simulink model "rule_intersection"  (R2021a)
settings: Solver=FixedStepAuto  StartTime=0.0  StopTime=47  FixedStep=0.1  RelTol=1e-3
values from neighbouring files (symbols this model uses):
  Cross =     [Cross.mat]
libraries: simulink x17
(part 2 of 2)

== matlab function rule_intersection/right of way/红灯右转路权监测/Enabled Subsystem/stage2/MATLAB Function1 ==
  data: Decision_A_x input; Decision_A_y input; Tgt input; y output; Ego input; Thetamin input; Thetamax input
function y = fcn(Decision_A_x,Decision_A_y,Tgt,Ego,Thetamin,Thetamax)
Tgtx = Tgt.TgtX;
Tgty = Tgt.TgtY;
Tgttheta = Tgt.Tgttheta;
Egovx = Ego.Egovx;
flag = (Tgttheta>Thetamin(1) & Tgttheta<Thetamax(1)) | (Tgttheta>Thetamin(2) & Tgttheta<Thetamax(2));
Tgtx = Tgtx.*flag;
Tgty = Tgty.*flag;
[in,~] = inpolygon(Tgtx,Tgty,Decision_A_x,Decision_A_y);

if sum(in)>0 && Egovx==0
    y = 1;
else
    y = 0;
end

== matlab function rule_intersection/right of way/左转路权监测/对向直行车道交点/rightarc_r ==
  data: u1 input; X output; u2 input; Y output; u4 input; u6 input
function [X,Y] = fcn(u1,u2,u4,u6)

locate_rf = [u1(7),u1(8)];
intention_rr = [u2(7),u2(8)];
r2l1_rf = [u4(5),u4(6)];
r4l_1_rr = [u6(7),u6(8)];
[x1,y1] = arc_generate_l(locate_rf(1),locate_rf(2),intention_rr(1),intention_rr(2));
for i = 1:19
    X1 = [x1(i),y1(i)]; X2 = [x1(i+1),y1(i+1)];
    [y,X,Y] = iscross(r2l1_rf,r4l_1_rr,X1,X2);
    if y == 1
        break
    end
end

== matlab function rule_intersection/right of way/左转路权监测/对向直行车道交点/MATLAB Function ==
  data: r_1r input; Intersect_A_x output; r_1l input; l_1r input; l_1l input; DPl input; DPr input; Intersect_A_y output; Decision_A_x output; Decision_A_y output
function [Intersect_A_x,Intersect_A_y,Decision_A_x,Decision_A_y] = fcn(r_1r,r_1l,l_1r,l_1l,DPl,DPr)

Intersect_A_x = [r_1r(1),r_1l(1),l_1l(1),l_1r(1),r_1r(1)];
Intersect_A_y = [r_1r(2),r_1l(2),l_1l(2),l_1r(2),r_1r(2)];
Decision_A_x = [l_1r(1),l_1l(1),DPl(1),DPr(1),l_1r(1)];
Decision_A_y = [l_1r(2),l_1l(2),DPl(2),DPr(2),l_1r(2)];

== matlab function rule_intersection/自车五个点 ==
  data: Ego input; X output; Y output
function [X,Y] = fcn(Ego)
Egox = Ego.EgoX;
Egoy = Ego.EgoY;
theta = Ego.Egotheta;
length = Ego.length;
width = Ego.width;
lf_x = Egox + 0.5*length*cos(theta) - 0.5*width*sin(theta);
lf_y = Egoy + 0.5*length*sin(theta) + 0.5*width*cos(theta);
lr_x = Egox - 0.5*length*cos(theta) - 0.5*width*sin(theta);
lr_y = Egoy - 0.5*length*sin(theta) + 0.5*width*cos(theta);
rf_x = Egox + 0.5*length*cos(theta) + 0.5*width*sin(theta);
rf_y = Egoy + 0.5*length*sin(theta) - 0.5*width*cos(theta);
rr_x = Egox - 0.5*length*cos(theta) + 0.5*width*sin(theta);
rr_y = Egoy - 0.5*length*sin(theta) - 0.5*width*cos(theta);
X = [Egox,lf_x,lr_x,rf_x,rr_x];
Y = [Egoy,lf_y,lr_y,rf_y,rr_y];

== matlab function rule_intersection/right of way/左转路权监测/MATLAB Function ==
  data: X input; t1 output; Y input; Intersect_A_x input; Intersect_A_y input; t2 output
function [t1,t2] = fcn(X,Y,Intersect_A_x,Intersect_A_y)
[in1,~] = inpolygon(X(1),Y(1),Intersect_A_x,Intersect_A_y);
[in2,~] = inpolygon(X(2),Y(2),Intersect_A_x,Intersect_A_y);
if ~in1 & in2  %驶入阶段
    t1 = 1;
    t2 = 0;
elseif in1  %通过阶段
    t1 = 0;
    t2 = 1;
else
    t1 = 0;
    t2 = 0;
end

== matlab function rule_intersection/right of way/Subsystem/MATLAB Function1 ==
  data: u input; y output
function y = fcn(u)

y = sign(u(1));

== matlab function rule_intersection/right of way/左转路权监测/输出对向方向预测线 ==
  data: u input; DPline output; Cross input; Theta_max output; Theta_min output
function [DPline,Theta_max,Theta_min] = fcn(u,Cross)

if u(1) == 1
    Zin = Cross.road3.zin;
    DPline = [Zin(1)+0,Zin(2),Zin(5)+0,Zin(6)];
    Theta_max = [15*pi/180,0];
    Theta_min = [0,-15*pi/180];
elseif u(1) == 2
    Zin = Cross.road4.zin;
    DPline = [Zin(1),Zin(2)+0,Zin(5),Zin(6)+0];
    Theta_max = [105*pi/180,90*pi/180];
    Theta_min = [90*pi/180,75*pi/180];
elseif u(1) == 3
    Zin = Cross.road1.zin;
    DPline = [Zin(1)-0,Zin(2),Zin(5)-0,Zin(6)];
    Theta_max = [pi,-165*pi/180];
    Theta_min = [165*pi/180,-pi];
else
    Zin = Cross.road2.zin;
    DPline = [Zin(1),Zin(2)-0,Zin(5),Zin(6)-0];
    Theta_max = [-75*pi/180,-90*pi/180];
    Theta_min = [-90*pi/180,-105*pi/180];
end

== matlab function rule_intersection/right of way/红灯右转路权监测/MATLAB Function ==
  data: X input; t1 output; Y input; Intersect_A_x input; Intersect_A_y input; t2 output
function [t1,t2] = fcn(X,Y,Intersect_A_x,Intersect_A_y)
[in1,~] = inpolygon(X(1),Y(1),Intersect_A_x,Intersect_A_y);
[in2,~] = inpolygon(X(2),Y(2),Intersect_A_x,Intersect_A_y);
if ~in1 & in2  %驶入阶段
    t1 = 1;
    t2 = 0;
elseif in1  %通过阶段
    t1 = 0;
    t2 = 1;
else
    t1 = 0;
    t2 = 0;
end

== matlab function rule_intersection/right of way/红灯右转路权监测/左侧直行车道交点/DPline_直行交点 ==
  data: u1 input; u3 input; u4 input; u5 input; u6 input; r2l1_DP_l output; u input; r2l1_DP_r output
function [r2l1_DP_l,r2l1_DP_r] = fcn(u1,u3,u4,u5,u6,u)

DPline_l = [u(1),u(2)];
DPline_r = [u(3),u(4)];

r2l1_lf = [u3(1),u3(2)];
r4l_1_lr = [u5(3),u5(4)];
r2l1_rf = [u4(5),u4(6)];
r4l_1_rr = [u6(7),u6(8)];
[~,Xl,Yl] = iscross(r2l1_lf,r4l_1_lr,DPline_l,DPline_r);
[~,Xr,Yr] = iscross(r2l1_rf,r4l_1_rr,DPline_l,DPline_r);
r2l1_DP_l = [Xl,Yl];
r2l1_DP_r = [Xr,Yr];

== matlab function rule_intersection/right of way/红灯右转路权监测/左侧直行车道交点/MATLAB Function ==
  data: r_r input; Intersect_A_x output; r_l input; l_r input; l_l input; DPl input; DPr input; Intersect_A_y output; Decision_A_x output; Decision_A_y output
function [Intersect_A_x,Intersect_A_y,Decision_A_x,Decision_A_y] = fcn(r_r,r_l,l_r,l_l,DPl,DPr)

Intersect_A_x = [r_r(1),r_l(1),l_l(1),l_r(1),r_r(1)];
Intersect_A_y = [r_r(2),r_l(2),l_l(2),l_r(2),r_r(2)];
Decision_A_x = [l_r(1),l_l(1),DPl(1),DPr(1),l_r(1)];
Decision_A_y = [l_r(2),l_l(2),DPl(2),DPr(2),l_r(2)];

== matlab function rule_intersection/right of way/红灯右转路权监测/左侧直行车道交点/leftarc_l ==
  data: u1 input; X output; u2 input; Y output; u3 input; u5 input
function [X,Y] = fcn(u1,u2,u3,u5)

locate_lf = [u1(3),u1(4)];
intention_lr = [u2(3),u2(4)];
r2l1_lf = [u3(1),u3(2)];
r4l_1_lr = [u5(3),u5(4)];
[x1,y1] = arc_generate_r(locate_lf(1),locate_lf(2),intention_lr(1),intention_lr(2));
x1 = [intention_lr(1),x1(2:end)];
y1 = [intention_lr(2),y1(2:end)];
for i = 1:19
    X1 = [x1(i),y1(i)]; X2 = [x1(i+1),y1(i+1)];
    [y,X,Y] = iscross(r2l1_lf,r4l_1_lr,X1,X2);
    if y == 1
        break
    end
end

== matlab function rule_intersection/right of way/左转路权监测/对向直行车道交点/DPline_直行交点 ==
  data: u1 input; u3 input; u4 input; u5 input; u6 input; r2l1_DP_l output; u input; r2l1_DP_r output
function [r2l1_DP_l,r2l1_DP_r] = fcn(u1,u3,u4,u5,u6,u)

DPline_l = [u(1),u(2)];
DPline_r = [u(3),u(4)];

r2l1_lf = [u3(1),u3(2)];
r4l_1_lr = [u5(3),u5(4)];
r2l1_rf = [u4(5),u4(6)];
r4l_1_rr = [u6(7),u6(8)];
[~,Xl,Yl] = iscross(r2l1_lf,r4l_1_lr,DPline_l,DPline_r);
[~,Xr,Yr] = iscross(r2l1_rf,r4l_1_rr,DPline_l,DPline_r);
r2l1_DP_l = [Xl,Yl];
r2l1_DP_r = [Xr,Yr];

== matlab function rule_intersection/right of way/红灯右转路权监测/左侧直行车道交点/leftarc_r ==
  data: u1 input; X output; u2 input; Y output; u4 input; u6 input
function [X,Y] = fcn(u1,u2,u4,u6)

locate_lf = [u1(3),u1(4)];
intention_lr = [u2(3),u2(4)];
r2l1_rf = [u4(5),u4(6)];
r4l_1_rr = [u6(7),u6(8)];
[x1,y1] = arc_generate_r(locate_lf(1),locate_lf(2),intention_lr(1),intention_lr(2));
for i = 1:19
    X1 = [x1(i),y1(i)]; X2 = [x1(i+1),y1(i+1)];
    [y,X,Y] = iscross(r2l1_rf,r4l_1_rr,X1,X2);
    if y == 1
        break
    end
end

== matlab function rule_intersection/right of way/左转路权监测/对向直行车道交点/rightarc_l ==
  data: u1 input; X output; u2 input; Y output; u3 input; u5 input
function [X,Y] = fcn(u1,u2,u3,u5)

locate_rf = [u1(7),u1(8)];
intention_rr = [u2(7),u2(8)];
r2l1_lf = [u3(1),u3(2)];
r4l_1_lr = [u5(3),u5(4)];
[x1,y1] = arc_generate_l(locate_rf(1),locate_rf(2),intention_rr(1),intention_rr(2));
for i = 1:19
    X1 = [x1(i),y1(i)]; X2 = [x1(i+1),y1(i+1)];
    [y,X,Y] = iscross(r2l1_lf,r4l_1_lr,X1,X2);
    if y == 1
        break
    end
end

== matlab function rule_intersection/right of way/左转路权监测/Enabled Subsystem/stage2/MATLAB Function1 ==
  data: Decision_A_x input; Decision_A_y input; Tgt input; y output; Ego input; Thetamin input; Thetamax input
function y = fcn(Decision_A_x,Decision_A_y,Tgt,Ego,Thetamin,Thetamax)
Tgtx = Tgt.TgtX;
Tgty = Tgt.TgtY;
Tgttheta = Tgt.Tgttheta;
Egovx = Ego.Egovx;
flag = (Tgttheta>Thetamin(1) & Tgttheta<Thetamax(1)) | (Tgttheta>Thetamin(2) & Tgttheta<Thetamax(2));
Tgtx = Tgtx.*flag;
Tgty = Tgty.*flag;
[in,~] = inpolygon(Tgtx,Tgty,Decision_A_x,Decision_A_y);

if sum(in)>0 && Egovx==0
    y = 1;
else
    y = 0;
end

== matlab function rule_intersection/right of way/红灯右转路权监测/左侧直行车道交点/rightarc_r ==
  data: u1 input; X output; u2 input; Y output; u4 input; u6 input
function [X,Y] = fcn(u1,u2,u4,u6)

locate_rf = [u1(7),u1(8)];
intention_rr = [u2(7),u2(8)];
r2l1_rf = [u4(5),u4(6)];
r4l_1_rr = [u6(7),u6(8)];
[x1,y1] = arc_generate_r(locate_rf(1),locate_rf(2),intention_rr(1),intention_rr(2));
for i = 1:19
    X1 = [x1(i),y1(i)]; X2 = [x1(i+1),y1(i+1)];
    [y,X,Y] = iscross(r2l1_rf,r4l_1_rr,X1,X2);
    if y == 1
        break
    end
end

== matlab function rule_intersection/right of way/红灯右转路权监测/输出左侧方向预测线 ==
  data: u input; DPline output; Cross input; Theta_max output; Theta_min output
function [DPline,Theta_max,Theta_min] = fcn(u,Cross)

if u(1) == 1
    Zin = Cross.road4.zin;
    DPline = [Zin(1),Zin(2)+2,Zin(5),Zin(6)+2];
    Theta_max = [105*pi/180,90*pi/180];
    Theta_min = [90*pi/180,75*pi/180];
elseif u(1) == 2
    Zin = Cross.road1.zin;
    DPline = [Zin(1)-2,Zin(2),Zin(5)-2,Zin(6)];
    Theta_max = [pi,-165*pi/180];
    Theta_min = [165*pi/180,-pi];
elseif u(1) == 3
    Zin = Cross.road2.zin;
    DPline = [Zin(1),Zin(2)-2,Zin(5),Zin(6)-2];
    Theta_max = [-75*pi/180,-90*pi/180];
    Theta_min = [-90*pi/180,-105*pi/180];
else
    Zin = Cross.road3.zin;
    DPline = [Zin(1)+2,Zin(2),Zin(5)+2,Zin(6)];
    Theta_max = [15*pi/180,0];
    Theta_min = [0,-15*pi/180];
end

== matlab function rule_intersection/right of way/输出红绿灯信息 ==
  data: u input; Light input; light output
function light = fcn(u,Light)


if u(1) == 1
    light = Light.light1;
elseif u(1) == 2
    light = Light.light2;
elseif u(1) == 3
    light = Light.light3;
elseif u(1) == 4
    light = Light.light4;
else
    light = 0;
end

== matlab function rule_intersection/right of way/绿灯右转路权监测/Enabled Subsystem/stage1/MATLAB Function2 ==
  data: ODA1 input; ODA2 input; Tgt input; y output; Ego input; Thetamin input; Thetamax input
function y = fcn(ODA1,ODA2,Tgt,Ego,Thetamin,Thetamax)
Tgtx = Tgt.TgtX;
Tgty = Tgt.TgtY;
Tgttheta = Tgt.Tgttheta;
Egovx = Ego.Egovx;
flag = (Tgttheta>Thetamin(1) & Tgttheta<Thetamax(1)) | (Tgttheta>Thetamin(2) & Tgttheta<Thetamax(2));
Tgtx = Tgtx.*flag;
Tgty = Tgty.*flag;
[in1,~] = inpolygon(Tgtx,Tgty,ODA1(1,:),ODA1(2,:));
[in2,~] = inpolygon(Tgtx,Tgty,ODA2(1,:),ODA2(2,:));
in = in1.*in2;

if sum(in)>0 && Egovx~=0
    y = 1;
else
    y = 0;
end

== matlab function rule_intersection/right of way/绿灯右转路权监测/Enabled Subsystem/stage2/MATLAB Function1 ==
  data: ODA1 input; ODA2 input; Tgt input; y output; Ego input; Thetamin input; Thetamax input
function y = fcn(ODA1,ODA2,Tgt,Ego,Thetamin,Thetamax)
Tgtx = Tgt.TgtX;
Tgty = Tgt.TgtY;
Tgttheta = Tgt.Tgttheta;
Egovx = Ego.Egovx;
flag = (Tgttheta>Thetamin(1) & Tgttheta<Thetamax(1)) | (Tgttheta>Thetamin(2) & Tgttheta<Thetamax(2));
Tgtx = Tgtx.*flag;
Tgty = Tgty.*flag;
[in1,~] = inpolygon(Tgtx,Tgty,ODA1(1,:),ODA1(2,:));
[in2,~] = inpolygon(Tgtx,Tgty,ODA2(1,:),ODA2(2,:));
in = in1.*in2;
if sum(in)>0 && Egovx==0
    y = 1;
else
    y = 0;
end

== matlab function rule_intersection/right of way/绿灯右转路权监测/MATLAB Function ==
  data: X input; t1 output; Y input; Intersect_A_x input; Intersect_A_y input; t2 output
function [t1,t2] = fcn(X,Y,Intersect_A_x,Intersect_A_y)
[in1,~] = inpolygon(X(1),Y(1),Intersect_A_x,Intersect_A_y);
[in2,~] = inpolygon((X(2)+X(3))/2,(Y(2)+Y(3))/2,Intersect_A_x,Intersect_A_y);
if ~in1 & in2  %驶入阶段
    t1 = 1;
    t2 = 0;
elseif in1  %通过阶段
    t1 = 0;
    t2 = 1;
else
    t1 = 0;
    t2 = 0;
end

== matlab function rule_intersection/right of way/绿灯右转路权监测/左侧直行车道交点/leftarc_l3 ==
  data: X output; arcx input; arcy input; Y output; u1 input; u2 input
function [X,Y] = fcn(arcx,arcy,u1,u2)
[x1,y1] = arc_generate_r(u1(3),u1(4),u2(3),u2(4));
y = 0;
for i = 1:19
    for j = 1:19
        X1 = [arcx(j),arcy(j)]; X2 = [arcx(j+1),arcy(j+1)];
        X3 = [x1(i),y1(i)]; X4 = [x1(i+1),y1(i+1)];
        [y,X,Y] = iscross(X1,X2,X3,X4);
        if y == 1
            break
        end
    end
    if y == 1
        break
    end
end

== matlab function rule_intersection/virtual lane/Subsystem/MATLAB Function1 ==
  data: u input; y output
function y = fcn(u)

y = sign(u(1));

== matlab function rule_intersection/right of way/绿灯右转路权监测/左侧直行车道交点/MATLAB Function1 ==
  data: u1 input; u2 output; OD_rarc_x output; OD_rarc_y output; ODA1 output; ODA2 output; DPline input
function [u2,OD_rarc_x,OD_rarc_y,ODA1,ODA2] = fcn(u1,DPline)
u2 = zeros(1,11);
u3 = zeros(1,11);
u4 = zeros(1,11);
OD_larc_x = zeros(1,20);
OD_larc_y = zeros(1,20);
OD_rarc_x = zeros(1,20);
OD_rarc_y = zeros(1,20);
coder.extrinsic('tright_G');
[u2,u3,u4] = tright_G(u1);
coder.extrinsic('arc_generate_l')
[OD_larc_x,OD_larc_y]=arc_generate_l(u3(1),u3(2),u2(3),u2(4));
[OD_rarc_x,OD_rarc_y]=arc_generate_l(u4(5),u4(6),u2(7),u2(8));
ODA1 = zeros(2,41);
ODA2 = zeros(2,4);
ODA1(1,:) = [OD_larc_x,fliplr(OD_rarc_x),OD_larc_x(1)];
ODA1(2,:) = [OD_larc_y,fliplr(OD_rarc_y),OD_larc_y(1)];
ODA2(1,:) = [DPline(1:2:5),DPline(1)];
ODA2(2,:) = [DPline(2:2:6),DPline(2)];

== matlab function rule_intersection/right of way/红灯右转路权监测/Enabled Subsystem/stage1/MATLAB Function2 ==
  data: Decision_A_x input; Decision_A_y input; Tgt input; y output; Ego input; Thetamin input; Thetamax input
function y = fcn(Decision_A_x,Decision_A_y,Tgt,Ego,Thetamin,Thetamax)
Tgtx = Tgt.TgtX;
Tgty = Tgt.TgtY;
Tgttheta = Tgt.Tgttheta;
Egovx = Ego.Egovx;
flag = (Tgttheta>Thetamin(1) & Tgttheta<Thetamax(1)) | (Tgttheta>Thetamin(2) & Tgttheta<Thetamax(2));
Tgtx = Tgtx.*flag;
Tgty = Tgty.*flag;
[in,~] = inpolygon(Tgtx,Tgty,Decision_A_x,Decision_A_y);

if sum(in)>0 && Egovx~=0
    y = 1;
else
    y = 0;
end

== matlab function rule_intersection/right of way/绿灯右转路权监测/左侧直行车道交点/int ==
  data: u1 input; u2 input; Intersect_A_x output; arcx input; arcy input; Intersect_A_y output
function [Intersect_A_x,Intersect_A_y] = fcn(u1,u2,arcx,arcy)
[x1,y1] = arc_generate_r(u1(3),u1(4),u2(3),u2(4));
y = 0;
for i = 1:19
    for j = 1:19
        X1 = [arcx(j),arcy(j)]; X2 = [arcx(j+1),arcy(j+1)];
        X3 = [x1(i),y1(i)]; X4 = [x1(i+1),y1(i+1)];
        [y,X,Y] = iscross(X1,X2,X3,X4);
        if y == 1
            break
        end
    end
    if y == 1
        break
    end
end
Intersect_A_x = [X,u2(3),u2(7),X];
Intersect_A_y = [Y,u2(4),u2(8),Y];

== matlab function rule_intersection/virtual lane/turn left/MATLAB Function3 ==
  data: u7 input; u8 input; u1 input; xl2 output; yl2 output; xr2 output; yr2 output
function [xl2,yl2,xr2,yr2] = fcn(u7,u8,u1)

locate_lf = [u1(3),u1(4)];
intention_lr = [u7(3),u7(4)];
locate_rf = [u1(7),u1(8)];
intention_rr = [u8(7),u8(8)];

[xl2,yl2] = arc_generate_l(locate_lf(1),locate_lf(2),intention_lr(1),intention_lr(2));
[xr2,yr2] = arc_generate_l(locate_rf(1),locate_rf(2),intention_rr(1),intention_rr(2));

== matlab function rule_intersection/virtual lane/turn right/MATLAB Function1 ==
  data: u1 input; xl output; u2 input; yl output; xr output; yr output
function [xl,yl,xr,yr] = fcn(u1,u2)

locate_lf = [u1(3),u1(4)];
intention_lr = [u2(3),u2(4)];
locate_rf = [u1(7),u1(8)];
intention_rr = [u2(7),u2(8)];

[xl,yl] = arc_generate_r(locate_lf(1),locate_lf(2),intention_lr(1),intention_lr(2));
[xr,yr] = arc_generate_r(locate_rf(1),locate_rf(2),intention_rr(1),intention_rr(2));

== matlab function rule_intersection/virtual lane/turn right/MATLAB Function2 ==
  data: xl input; yl input; xr input; y output; yr input; X input; Y input; xl2 input; yl2 input; xr2 input; yr2 input
function y = fcn(xl,yl,xr,yr,X,Y,xl2,yl2,xr2,yr2)
Decision_A_x = [xl,fliplr(xr),xl(1)];
Decision_A_y = [yl,fliplr(yr),yl(1)];
[in1,~] = inpolygon(X(1),Y(1),Decision_A_x,Decision_A_y);
Not_recommended_A_x = [xl2,fliplr(xr2),xl2(1)];
Not_recommended_A_y = [yl2,fliplr(yr2),yl2(1)];
[in2,~] = inpolygon(X(1),Y(1),Not_recommended_A_x,Not_recommended_A_y);
if in1
    y = 0;
elseif ~in1 && in2
    y = 2;  %不推荐
else
    y = 1;
end

== matlab function rule_intersection/right of way/红灯右转路权监测/左侧直行车道交点/MATLAB Function1 ==
  data: u1 input; u2 output; u3 output; u4 output; u5 output; u6 output
function [u2,u3,u4,u5,u6] = fcn(u1)
u2 = zeros(1,11);
u3 = zeros(1,11);
u4 = zeros(1,11);
u5 = zeros(1,11);
u6 = zeros(1,11);
coder.extrinsic('tright');
[u2,u3,u4,u5,u6] = tright(u1);

== matlab function rule_intersection/right of way/红灯右转路权监测/左侧直行车道交点/rightarc_l ==
  data: X output; Y output; u6 input
function [X,Y] = fcn(u6)
X = u6(7);
Y = u6(8);

== matlab function rule_intersection/right of way/绿灯右转路权监测/输出左侧方向预测线 ==
  data: u input; DPline output; Cross input; Theta_max output; Theta_min output
function [DPline,Theta_max,Theta_min] = fcn(u,Cross)
A1 = [Cross.road1.stop(1),Cross.road1.stop(2)];
A2 = [Cross.road1.stop(5),Cross.road1.stop(6)];
C1 = [Cross.road2.stop(1),Cross.road2.stop(2)];
C2 = [Cross.road2.stop(5),Cross.road2.stop(6)];
D1 = [Cross.road3.stop(1),Cross.road3.stop(2)];
D2 = [Cross.road3.stop(5),Cross.road3.stop(6)];
E1 = [Cross.road4.stop(1),Cross.road4.stop(2)];
E2 = [Cross.road4.stop(5),Cross.road4.stop(6)];
[x1,y1] = node(A1,A2,C1,C2);
[x2,y2] = node(C1,C2,D1,D2);
[x3,y3] = node(D1,D2,E1,E2);
[x4,y4] = node(E1,E2,A1,A2);

if u(1) == 1
    DPline = [x2,y2,x4,y4,x1,y1];
    Theta_max = [90*pi/180,45*pi/180];
    Theta_min = [45*pi/180,0*pi/180];
elseif u(1) == 2
    DPline = [x1,y1,x3,y3,x2,y2];
    Theta_max = [135*pi/180,180*pi/180];
    Theta_min = [90*pi/180,135*pi/180];
elseif u(1) == 3
    DPline = [x2,y2,x4,y4,x3,y3];
    Theta_max = [-90*pi/180,-135*pi/180];
    Theta_min = [-135*pi/180,-180*pi/180];
else
    DPline = [x1,y1,x3,y3,x4,y4];
    Theta_max = [0*pi/180,-45*pi/180];
    Theta_min = [-45*pi/180,-90*pi/180];
end

== matlab function rule_intersection/stop line/MATLAB Function ==
  data: u input; y output
function y = fcn(u)

y = u(1);

== matlab function rule_intersection/impede pedesrtain/Enabled Subsystem2/MATLAB Function ==
  data: c input; Cross input; y output; Ped input; X input; Y input
function y = fcn(c,Cross,Ped,X,Y)
coder.extrinsic('fieldnames')
number = 0;
number = length(unique(fieldnames(Cross.road1)));
number = number-3;
x_c = linspace(c(1,4),c(1,3),number+1);
C = zeros(number,10);
for i = 1:number
    C(i,:) = [x_c(i),x_c(i+1),x_c(i+1),x_c(i),x_c(i),c(2,1),c(2,1),c(2,4),c(2,4),c(2,1)];
end
x_f = (X(2)+X(4))/2;
y_f = (Y(2)+Y(4))/2;
px = Ped.PX;
py = Ped.PY;
pvx = Ped.Pvx;
pvy = Ped.Pvy;
tc1 = 0;
for i = 1:number
    [in1,~] = inpolygon(X(1),Y(1),C(i,1:5),C(i,6:10));
    [in2,~] = inpolygon(x_f,y_f,C(i,1:5),C(i,6:10));
    if ~in1 & in2  %驶入阶段
        tc1 = i;
        break;
    else
        tc1 = 0;
    end
end

if tc1 > 0 
    if tc1 == 1
        [In1,~] = inpolygon(px,py,C(tc1,1:5),C(tc1,6:10));
        [In2,~] = inpolygon(px,py,C(tc1+1,1:5),C(tc1+1,6:10));
        f1 = pvx>0.6;
        if sum(In1 |(In2 & f1))
            y = 1;
        else
            y = 0;
        end
    elseif tc1 == number
        [In1,~] = inpolygon(px,py,C(tc1,1:5),C(tc1,6:10));
        [In2,~] = inpolygon(px,py,C(tc1-1,1:5),C(tc1-1,6:10));
        f1 = pvx<-0.6;
        if sum(In1 |(In2 & f1))
            y = 1;
        else
            y = 0;
        end
    else
        [In1,~] = inpolygon(px,py,C(tc1,1:5),C(tc1,6:10));
        [In2,~] = inpolygon(px,py,C(tc1-1,1:5),C(tc1-1,6:10));
        f1 = pvx<-0.6;
        [In3,~] = inpolygon(px,py,C(tc1+1,1:5),C(tc1+1,6:10));
        f2 = pvx>0.6;
        if sum(In1 |(In2 & f1)|(In3 & f2))
            y = 1;
        else
            y = 0;
        end
    end
else
    y = 0;
end

== matlab function rule_intersection/impede pedesrtain/MATLAB Function ==
  data: X input; tc1 output; Y input; c1 input; c2 input; c3 input; c4 input; tc2 output; tc3 output; tc4 output
function [tc1,tc2,tc3,tc4] = fcn(X,Y,c1,c2,c3,c4)

x_f = (X(2)+X(4))/2;
y_f = (Y(2)+Y(4))/2;
[in1,~] = inpolygon(X(1),Y(1),c1(1,:),c1(2,:));
[in2,~] = inpolygon(x_f,y_f,c1(1,:),c1(2,:));
[in3,~] = inpolygon(X(1),Y(1),c2(1,:),c2(2,:));
[in4,~] = inpolygon(x_f,y_f,c2(1,:),c2(2,:));
[in5,~] = inpolygon(X(1),Y(1),c3(1,:),c3(2,:));
[in6,~] = inpolygon(x_f,y_f,c3(1,:),c3(2,:));
[in7,~] = inpolygon(X(1),Y(1),c4(1,:),c4(2,:));
[in8,~] = inpolygon(x_f,y_f,c4(1,:),c4(2,:));
if ~in1 & in2  %驶入阶段
    tc1 = 1;
else
    tc1 = 0;
end
if ~in3 & in4  %驶入阶段
    tc2 = 1;
else
    tc2 = 0;
end
if ~in5 & in6  %驶入阶段
    tc3 = 1;
else
    tc3 = 0;
end
if ~in7 & in8  %驶入阶段
    tc4 = 1;
else
    tc4 = 0;
end

== matlab function rule_intersection/stop on sidewalk/MATLAB Function ==
  data: Cross input; y output
function y = fcn(Cross)
coder.extrinsic('fieldnames')
y = 0;
y = length(unique(fieldnames(Cross.road1)));

== matlab function rule_intersection/所属车道计算 ==
  data: Ego input; road output; lane output; P output
function [road,lane,P] = fcn(Ego)
X = Ego.EgoX;
Y = Ego.EgoY;

coder.extrinsic('locate');
[r,l,p] = locate(X,Y);
road = 0;
road = r;
lane = 0;
lane = l;
P = zeros(1,11);
P =p;

== matlab function rule_intersection/impede pedesrtain/Enabled Subsystem1/MATLAB Function ==
  data: c input; Cross input; y output; Ped input; X input; Y input
function y = fcn(c,Cross,Ped,X,Y)
coder.extrinsic('fieldnames')
number = 0;
number = length(unique(fieldnames(Cross.road1)));
number = number-3;
y_c = linspace(c(2,4),c(2,3),number+1);
C = zeros(number,10);
for i = 1:number
    C(i,:) = [c(1,1),c(1,1),c(1,4),c(1,4),c(1,1),y_c(i),y_c(i+1),y_c(i+1),y_c(i),y_c(i)];
end
x_f = (X(2)+X(4))/2;
y_f = (Y(2)+Y(4))/2;
px = Ped.PX;
py = Ped.PY;
pvx = Ped.Pvx;
pvy = Ped.Pvy;
tc1 = 0;
for i = 1:number
    [in1,~] = inpolygon(X(1),Y(1),C(i,1:5),C(i,6:10));
    [in2,~] = inpolygon(x_f,y_f,C(i,1:5),C(i,6:10));
    if ~in1 & in2  %驶入阶段
        tc1 = i;
        break;
    else
        tc1 = 0;
    end
end

if tc1 > 0 
    if tc1 == 1
        [In1,~] = inpolygon(px,py,C(tc1,1:5),C(tc1,6:10));
        [In2,~] = inpolygon(px,py,C(tc1+1,1:5),C(tc1+1,6:10));
        f1 = pvy<-0.6;
        if sum(In1 |(In2 & f1))
            y = 1;
        else
            y = 0;
        end
    elseif tc1 == number
        [In1,~] = inpolygon(px,py,C(tc1,1:5),C(tc1,6:10));
        [In2,~] = inpolygon(px,py,C(tc1-1,1:5),C(tc1-1,6:10));
        f1 = pvy>0.6;
        if sum(In1 |(In2 & f1))
            y = 1;
        else
            y = 0;
        end
    else
        [In1,~] = inpolygon(px,py,C(tc1,1:5),C(tc1,6:10));
        [In2,~] = inpolygon(px,py,C(tc1-1,1:5),C(tc1-1,6:10));
        f1 = pvy>0.6;
        [In3,~] = inpolygon(px,py,C(tc1+1,1:5),C(tc1+1,6:10));
        f2 = pvy<-0.6;
        if sum(In1 |(In2 & f1)|(In3 & f2))
            y = 1;
        else
            y = 0;
        end
    end
else
    y = 0;
end

== matlab function rule_intersection/impede pedesrtain/Enabled Subsystem3/MATLAB Function ==
  data: c input; Cross input; y output; Ped input; X input; Y input
function y = fcn(c,Cross,Ped,X,Y)
coder.extrinsic('fieldnames')
number = 0;
number = length(unique(fieldnames(Cross.road1)));
number = number-3;
y_c = linspace(c(2,4),c(2,3),number+1);
C = zeros(number,10);
for i = 1:number
    C(i,:) = [c(1,1),c(1,1),c(1,4),c(1,4),c(1,1),y_c(i),y_c(i+1),y_c(i+1),y_c(i),y_c(i)];
end
x_f = (X(2)+X(4))/2;
y_f = (Y(2)+Y(4))/2;
px = Ped.PX;
py = Ped.PY;
pvx = Ped.Pvx;
pvy = Ped.Pvy;
tc1 = 0;
for i = 1:number
    [in1,~] = inpolygon(X(1),Y(1),C(i,1:5),C(i,6:10));
    [in2,~] = inpolygon(x_f,y_f,C(i,1:5),C(i,6:10));
    if ~in1 & in2  %驶入阶段
        tc1 = i;
        break;
    else
        tc1 = 0;
    end
end

if tc1 > 0 
    if tc1 == 1
        [In1,~] = inpolygon(px,py,C(tc1,1:5),C(tc1,6:10));
        [In2,~] = inpolygon(px,py,C(tc1+1,1:5),C(tc1+1,6:10));
        f1 = pvy>0.6;
        if sum(In1 |(In2 & f1))
            y = 1;
        else
            y = 0;
        end
    elseif tc1 == number
        [In1,~] = inpolygon(px,py,C(tc1,1:5),C(tc1,6:10));
        [In2,~] = inpolygon(px,py,C(tc1-1,1:5),C(tc1-1,6:10));
        f1 = pvy<-0.6;
        if sum(In1 |(In2 & f1))
            y = 1;
        else
            y = 0;
        end
    else
        [In1,~] = inpolygon(px,py,C(tc1,1:5),C(tc1,6:10));
        [In2,~] = inpolygon(px,py,C(tc1-1,1:5),C(tc1-1,6:10));
        f1 = pvy<-0.6;
        [In3,~] = inpolygon(px,py,C(tc1+1,1:5),C(tc1+1,6:10));
        f2 = pvy>0.6;
        if sum(In1 |(In2 & f1)|(In3 & f2))
            y = 1;
        else
            y = 0;
        end
    end
else
    y = 0;
end

== matlab function rule_intersection/impede pedesrtain/Enabled Subsystem4/MATLAB Function ==
  data: c input; Cross input; y output; Ped input; X input; Y input
function y = fcn(c,Cross,Ped,X,Y)
coder.extrinsic('fieldnames')
number = 0;
number = length(unique(fieldnames(Cross.road1)));
number = number-3;
x_c = linspace(c(1,4),c(1,3),number+1);
C = zeros(number,10);
for i = 1:number
    C(i,:) = [x_c(i),x_c(i+1),x_c(i+1),x_c(i),x_c(i),c(2,1),c(2,1),c(2,4),c(2,4),c(2,1)];
end
x_f = (X(2)+X(4))/2;
y_f = (Y(2)+Y(4))/2;
px = Ped.PX;
py = Ped.PY;
pvx = Ped.Pvx;
pvy = Ped.Pvy;
tc1 = 0;
for i = 1:number
    [in1,~] = inpolygon(X(1),Y(1),C(i,1:5),C(i,6:10));
    [in2,~] = inpolygon(x_f,y_f,C(i,1:5),C(i,6:10));
    if ~in1 & in2  %驶入阶段
        tc1 = i;
        break;
    else
        tc1 = 0;
    end
end

if tc1 > 0 
    if tc1 == 1
        [In1,~] = inpolygon(px,py,C(tc1,1:5),C(tc1,6:10));
        [In2,~] = inpolygon(px,py,C(tc1+1,1:5),C(tc1+1,6:10));
        f1 = pvx<-0.6;
        if sum(In1 |(In2 & f1))
            y = 1;
        else
            y = 0;
        end
    elseif tc1 == number
        [In1,~] = inpolygon(px,py,C(tc1,1:5),C(tc1,6:10));
        [In2,~] = inpolygon(px,py,C(tc1-1,1:5),C(tc1-1,6:10));
        f1 = pvx>0.6;
        if sum(In1 |(In2 & f1))
            y = 1;
        else
            y = 0;
        end
    else
        [In1,~] = inpolygon(px,py,C(tc1,1:5),C(tc1,6:10));
        [In2,~] = inpolygon(px,py,C(tc1-1,1:5),C(tc1-1,6:10));
        f1 = pvx>0.6;
        [In3,~] = inpolygon(px,py,C(tc1+1,1:5),C(tc1+1,6:10));
        f2 = pvx<-0.6;
        if sum(In1 |(In2 & f1)|(In3 & f2))
            y = 1;
        else
            y = 0;
        end
    end
else
    y = 0;
end

== matlab function rule_intersection/right of way/绿灯右转路权监测/左侧直行车道交点/leftarc_l1 ==
  data: X output; arcx input; arcy input; Y output; DPline input
function [X,Y] = fcn(arcx,arcy,DPline)
X = zeros(1,20);
y = zeros(1,20);
for i = 1:19
    X1 = [arcx(i),arcy(i)]; X2 = [arcx(i+1),arcy(i+1)];
    [y,X,Y] = iscross([DPline(1),DPline(2)],[DPline(3),DPline(4)],X1,X2);
    next = i+1;
    if y == 1
        break
    end
end
X(next-1) = x;
Y(next-1) = y;
for j = next:20
    X(j) = arcx(j);
    Y(j) = arcy(j);
end

== matlab function rule_intersection/right of way/绿灯右转路权监测/左侧直行车道交点/leftarc_l2 ==
  data: X output; arcx input; arcy input; Y output; DPline input
function [X,Y] = fcn(arcx,arcy,DPline)
X = zeros(1,20);
y = zeros(1,20);
for i = 1:19
    X1 = [arcx(i),arcy(i)]; X2 = [arcx(i+1),arcy(i+1)];
    [y2,x,y] = iscross([DPline(1),DPline(2)],[DPline(3),DPline(4)],X1,X2);
    next = i+1;
    if y2 == 1
        break
    end
end
X(next-1) = x;
Y(next-1) = y;
for j = next:20
    X(j) = arcx(j);
    Y(j) = arcy(j);
end

== matlab function rule_intersection/virtual lane/turn right/MATLAB Function3 ==
  data: u7 input; u8 input; u1 input; xl2 output; yl2 output; xr2 output; yr2 output
function [xl2,yl2,xr2,yr2] = fcn(u7,u8,u1)

locate_lf = [u1(3),u1(4)];
intention_lr = [u7(3),u7(4)];
locate_rf = [u1(7),u1(8)];
intention_rr = [u8(7),u8(8)];

[xl2,yl2] = arc_generate_r(locate_lf(1),locate_lf(2),intention_lr(1),intention_lr(2));
[xr2,yr2] = arc_generate_r(locate_rf(1),locate_rf(2),intention_rr(1),intention_rr(2));

== matlab function rule_intersection/virtual lane/turn right/目标车道 ==
  data: u1 input; u2 output; u7 output; u8 output
function [u2,u7,u8]  = fcn(u1)
u2 = zeros(1,11);
u7 = zeros(1,11);
u8 = zeros(1,11);
coder.extrinsic('tright');
[u2,~,~,~,~,u7,u8] = tright(u1);

== matlab function rule_intersection/virtual lane/go straight/MATLAB Function1 ==
  data: u1 input; xl output; u2 input; yl output; xr output; yr output
function [xl,yl,xr,yr] = fcn(u1,u2)

locate_lf = [u1(3),u1(4)];
intention_lr = [u2(3),u2(4)];
locate_rf = [u1(7),u1(8)];
intention_rr = [u2(7),u2(8)];
xl = [locate_lf(1),intention_lr(1)];
yl = [locate_lf(2),intention_lr(2)];
xr = [locate_rf(1),intention_rr(1)];
yr = [locate_rf(2),intention_rr(2)];

== matlab function rule_intersection/virtual lane/go straight/MATLAB Function2 ==
  data: xl input; yl input; xr input; y output; yr input; X input; Y input; xl2 input; yl2 input; xr2 input; yr2 input
function y = fcn(xl,yl,xr,yr,X,Y,xl2,yl2,xr2,yr2)
Decision_A_x = [xl,fliplr(xr),xl(1)];
Decision_A_y = [yl,fliplr(yr),yl(1)];
[in1,~] = inpolygon(X(1),Y(1),Decision_A_x,Decision_A_y);
Not_recommended_A_x = [xl2,fliplr(xr2),xl2(1)];
Not_recommended_A_y = [yl2,fliplr(yr2),yl2(1)];
[in2,~] = inpolygon(X(1),Y(1),Not_recommended_A_x,Not_recommended_A_y);
if in1
    y = 0;
elseif ~in1 && in2
    y = 2;  %不推荐
else
    y = 1;
end

== matlab function rule_intersection/right of way/左转路权监测/对向直行车道交点/MATLAB Function1 ==
  data: u1 input; u2 output; u3 output; u4 output; u5 output; u6 output
function [u2,u3,u4,u5,u6] = fcn(u1)
u2 = zeros(1,11);
u3 = zeros(1,11);
u4 = zeros(1,11);
u5 = zeros(1,11);
u6 = zeros(1,11);
coder.extrinsic('tleft');
[u2,u3,u4,u5,u6] = tleft(u1);

== matlab function rule_intersection/virtual lane/go straight/MATLAB Function3 ==
  data: u7 input; u8 input; u1 input; xl2 output; yl2 output; xr2 output; yr2 output
function [xl2,yl2,xr2,yr2] = fcn(u7,u8,u1)

locate_lf = [u1(3),u1(4)];
intention_lr = [u7(3),u7(4)];
locate_rf = [u1(7),u1(8)];
intention_rr = [u8(7),u8(8)];
xl2 = [locate_lf(1),intention_lr(1)];
yl2 = [locate_lf(2),intention_lr(2)];
xr2 = [locate_rf(1),intention_rr(1)];
yr2 = [locate_rf(2),intention_rr(2)];

== matlab function rule_intersection/virtual lane/go straight/目标车道 ==
  data: u1 input; u2 output; u3 output; u4 output
function [u2,u3,u4]  = fcn(u1)
u2 = zeros(1,11);
u3 = zeros(1,11);
u4 = zeros(1,11);
coder.extrinsic('gostright');
[u2,u3,u4] = gostright(u1);

== matlab function rule_intersection/stop on sidewalk/四个斑马线区域 ==
  data: cross input; c1 output; c2 output; c3 output; c4 output
%返回四个人行横道区域
%返回值：[x1, y1, x2, y2] 
%人行横道左上角x1坐标，人行横道左上角y1坐标
%人行横道右下角x2坐标，人行横道右下角y2坐标
function [c1, c2, c3, c4] = fcn(cross)
c1 = [cross.road1.zin(5), cross.road1.zin(6), cross.road1.zout(1), cross.road1.zin(2)];
c2 = [cross.road2.zin(5), cross.road2.zout(6), cross.road2.zin(1), cross.road2.zin(2)];
c3 = [cross.road3.zout(1), cross.road3.zin(2), cross.road3.zin(1), cross.road3.zin(6)];
c4 = [cross.road4.zin(1), cross.road4.zin(2), cross.road4.zin(5), cross.road3.zin(6)];

== matlab function rule_intersection/virtual lane/turn left/目标车道 ==
  data: u1 input; u2 output; u7 output; u8 output
function [u2,u7,u8]  = fcn(u1)
u2 = zeros(1,11);
u7 = zeros(1,11);
u8 = zeros(1,11);
coder.extrinsic('tleft');
[u2,~,~,~,~,u7,u8] = tleft(u1);

== matlab function rule_intersection/stop on sidewalk/速度,相交前车判断 ==
  data: c1 input; enable output; c2 input; c3 input; c4 input; X input; Y input; EGO input
%判断是否与斑马线区域重叠且速度为零
function enable = fcn(c1, c2, c3, c4, X, Y, EGO)

coder.extrinsic('isoverlap');

EgoInfo = [X(2), Y(2), X(5), Y(5)];

overlap = isoverlap(EgoInfo, c1) && isoverlap(EgoInfo, c2) && isoverlap(EgoInfo, c3) && isoverlap(EgoInfo, c4);

static = EGO.Egovx == 0 && EGO.Egovy == 0;

enable = static && overlap;

== matlab function rule_intersection/stop line/Subsystem/MATLAB Function1 ==
  data: u input; y output
function y = fcn(u)

y = sign(u(1));

== matlab function rule_intersection/stop line/停车线坐标 ==
  data: location input; s1 output; cross input; s2 output
function [s1, s2] = fcn(location, cross)

switch  location(1)
    case 0
        s1 = [0,0,0];
        s2 = [0,0,0];
    case 1
        s1 = [cross.road1.stop(1), cross.road1.stop(2), 0];
        s2 = [cross.road1.stop(5), cross.road1.stop(6), 0];
    case 2
        s1 = [cross.road2.stop(1), cross.road2.stop(2), 0];
        s2 = [cross.road2.stop(5), cross.road2.stop(6), 0];
    case 3
        s1 = [cross.road3.stop(1), cross.road3.stop(2), 0];
        s2 = [cross.road3.stop(5), cross.road3.stop(6), 0];
    case 4
        s1 = [cross.road4.stop(1), cross.road4.stop(2), 0];
        s2 = [cross.road4.stop(5), cross.road4.stop(6), 0];
    otherwise
        s1 = [0,0,0];
        s2 = [0,0,0];
end

== matlab function rule_intersection/stop line/判断是否接近路口 ==
  data: location input; S1 input; S2 input; trigger output; X input; Y input; distance output
function [trigger,distance] = fcn(location, S1, S2, X, Y)

coder.extrinsic('point2line');
EgoPos = [X(1), Y(1), 0];

if location(1) == 0
    distance = 0;
else 
    distance = point2line(EgoPos, S1, S2);
end
    
if distance <= 5
    trigger = 1;
else
    trigger = 0;
end

== matlab function rule_intersection/stop line/开始进行停车线判断/红灯通行规则/Triggered Subsystem/判断自车变红灯时初始位置 ==
  data: red_enable output; location_flag input; trigger output
%

function [red_enable, trigger]= fcn(location_flag)
if location_flag == 0 %before entering the crossroad
    trigger = 1;
    red_enable = 0;
else
    trigger = 0;
    red_enable = 1;
end

== matlab function rule_intersection/stop line/开始进行停车线判断/红灯通行规则/右转? ==
  data: Ego input; pass output; enable output
%判断是否为右转
%如右转，pass = 1
%其余情况 trigger = 1, pass = 0
function [pass, enable] = fcn(Ego)

Decision = Ego.Decision;

if Decision == 2
    pass = 1;
    enable = 0;
else
    pass = 0;
    enable = 1;
end

== matlab function rule_intersection/right of way/左转路权监测/对向直行车道交点/leftarc_l ==
  data: u1 input; X output; u2 input; Y output; u3 input; u5 input
function [X,Y] = fcn(u1,u2,u3,u5)

locate_lf = [u1(3),u1(4)];
intention_lr = [u2(3),u2(4)];
r2l1_lf = [u3(1),u3(2)];
r4l_1_lr = [u5(3),u5(4)];
[x1,y1] = arc_generate_l(locate_lf(1),locate_lf(2),intention_lr(1),intention_lr(2));
for i = 1:19
    X1 = [x1(i),y1(i)]; X2 = [x1(i+1),y1(i+1)];
    [y,X,Y] = iscross(r2l1_lf,r4l_1_lr,X1,X2);
    if y == 1
        break
    end
end

== matlab function rule_intersection/stop line/开始进行停车线判断/触碰停止线/MATLAB Function ==
  data: touch output; X input; Y input; S1 input; S2 input
%通过判断车右前侧和右后侧连线是否与停止线相交来判断是否越过停止线

function touch = fcn(X, Y, S1, S2)
coder.extrinsic('iscross');
y = zeros(1);
Px = zeros(1);
Py = zeros(1);
[y, Px, Py] = iscross([X(4),Y(4)], [X(5),Y(5)], S1(1:2), S2(1:2));

if y == 1 
    touch = 1;
else 
    touch = 0;
end

== matlab function rule_intersection/stop line/开始进行停车线判断/黄灯通行规则/判断是否pass stopline ==
  data: Ego input; X input; pass output; Y input; S1 input; S2 input; enable output
%通过判断车右前侧和右后侧连线是否与停止线相交来判断是否越过停止线

function [pass, enable] = fcn(Ego, X, Y, S1, S2)
coder.extrinsic('iscross');
y = zeros(1);
Px = zeros(1);
Py = zeros(1);
[y, Px, Py] = iscross([X(4),Y(4)], [X(5),Y(5)], S1(1:2), S2(1:2));

if y == 1 && Ego.Egovx ~= 0
    pass = 1;
   enable = 0;
else 
    pass = 0;
    enable = 1;
end

== matlab function rule_intersection/stop line/输出红绿灯信息 ==
  data: u input; Light input; light output
function light = fcn(u,Light)


if u(1) == 1
    light = Light.light1;
elseif u(1) == 2
    light = Light.light2;
elseif u(1) == 3
    light = Light.light3;
elseif u(1) == 4
    light = Light.light4;
else
    light = 0;
end

== matlab function rule_intersection/virtual lane/turn left/MATLAB Function1 ==
  data: u1 input; xl output; u2 input; yl output; xr output; yr output
function [xl,yl,xr,yr] = fcn(u1,u2)

locate_lf = [u1(3),u1(4)];
intention_lr = [u2(3),u2(4)];
locate_rf = [u1(7),u1(8)];
intention_rr = [u2(7),u2(8)];

[xl,yl] = arc_generate_l(locate_lf(1),locate_lf(2),intention_lr(1),intention_lr(2));
[xr,yr] = arc_generate_l(locate_rf(1),locate_rf(2),intention_rr(1),intention_rr(2));

== matlab function rule_intersection/virtual lane/turn left/MATLAB Function2 ==
  data: xl input; yl input; xr input; y output; yr input; X input; Y input; xl2 input; yl2 input; xr2 input; yr2 input
function y = fcn(xl,yl,xr,yr,X,Y,xl2,yl2,xr2,yr2)
Decision_A_x = [xl,fliplr(xr),xl(1)];
Decision_A_y = [yl,fliplr(yr),yl(1)];
[in1,~] = inpolygon(X(1),Y(1),Decision_A_x,Decision_A_y);
Not_recommended_A_x = [xl2,fliplr(xr2),xl2(1)];
Not_recommended_A_y = [yl2,fliplr(yr2),yl2(1)];
[in2,~] = inpolygon(X(1),Y(1),Not_recommended_A_x,Not_recommended_A_y);
if in1
    y = 0;
elseif ~in1 && in2
    y = 2;  %不推荐
else
    y = 1;
end

== matlab function rule_intersection/impede pedesrtain/四个斑马线区域 ==
  data: cross input; c1 output; c2 output; c3 output; c4 output
%返回四个人行横道区域

function [c1, c2, c3, c4] = fcn(cross)

c1 = [cross.road1.zin(1), cross.road1.zin(5),cross.road1.zout(5),cross.road1.zout(1),cross.road1.zin(1); cross.road1.zin(2), cross.road1.zin(6), cross.road1.zout(6),  cross.road1.zout(2), cross.road1.zin(2)];
c2 = [cross.road2.zin(1), cross.road2.zin(5),cross.road2.zout(5),cross.road2.zout(1),cross.road2.zin(1); cross.road2.zin(2), cross.road2.zin(6), cross.road2.zout(6),  cross.road2.zout(2), cross.road2.zin(2)];
c3 = [cross.road3.zin(1), cross.road3.zin(5),cross.road3.zout(5),cross.road3.zout(1),cross.road3.zin(1); cross.road3.zin(2), cross.road3.zin(6), cross.road3.zout(6),  cross.road3.zout(2), cross.road3.zin(2)];
c4 = [cross.road4.zin(1), cross.road4.zin(5),cross.road4.zout(5),cross.road4.zout(1),cross.road4.zin(1); cross.road4.zin(2), cross.road4.zin(6), cross.road4.zout(6),  cross.road4.zout(2), cross.road4.zin(2)];

== matlab function rule_intersection/right of way/左转路权监测/对向直行车道交点/leftarc_r ==
  data: u1 input; X output; u2 input; Y output; u4 input; u6 input
function [X,Y] = fcn(u1,u2,u4,u6)

locate_lf = [u1(3),u1(4)];
intention_lr = [u2(3),u2(4)];
r2l1_rf = [u4(5),u4(6)];
r4l_1_rr = [u6(7),u6(8)];
[x1,y1] = arc_generate_l(locate_lf(1),locate_lf(2),intention_lr(1),intention_lr(2));
for i = 1:19
    X1 = [x1(i),y1(i)]; X2 = [x1(i+1),y1(i+1)];
    [y,X,Y] = iscross(r2l1_rf,r4l_1_rr,X1,X2);
    if y == 1
        break
    end
end

== matlab function rule_intersection/right of way/左转路权监测/Enabled Subsystem/stage1/MATLAB Function2 ==
  data: Decision_A_x input; Decision_A_y input; Tgt input; y output; Ego input; Thetamin input; Thetamax input
function y = fcn(Decision_A_x,Decision_A_y,Tgt,Ego,Thetamin,Thetamax)
Tgtx = Tgt.TgtX;
Tgty = Tgt.TgtY;
Tgttheta = Tgt.Tgttheta;
Egovx = Ego.Egovx;
flag = (Tgttheta>Thetamin(1) & Tgttheta<Thetamax(1)) | (Tgttheta>Thetamin(2) & Tgttheta<Thetamax(2));
Tgtx = Tgtx.*flag;
Tgty = Tgty.*flag;
[in,~] = inpolygon(Tgtx,Tgty,Decision_A_x,Decision_A_y);
if sum(in)>0 && Egovx~=0
    y = 1;
else
    y = 0;
end
